simulink model "RoboticsCoursework2"  (R2018b)
settings: Solver=ode4  StartTime=0.0  StopTime=5.0  FixedStep=0.005  RelTol=1e-3
undefined symbols (not defined in the file or in its folder): p560
libraries: roblocks x4
settings Model: Creator=57035  LastModifiedBy=57035

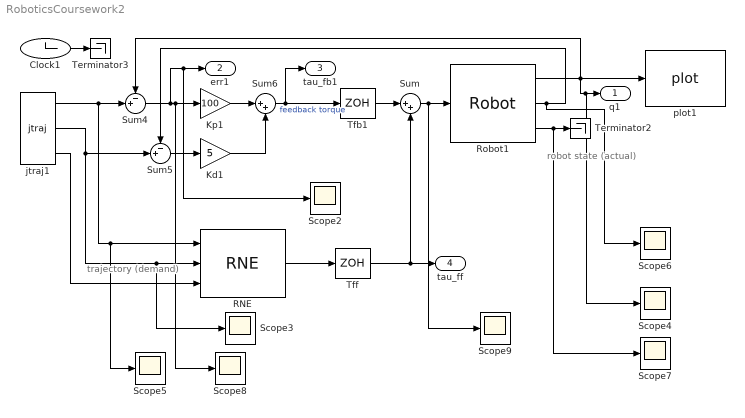
== system RoboticsCoursework2 ==
  note: trajectory
      | (demand)
  note: robot state
      | (actual)
  Clock1 : Clock
  Kd1 : Gain  Gain=5  SaturateOnIntegerOverflow=on  OutDataTypeStr=Inherit: Same as input  ParamDataTypeStr=Inherit: Same as input
  Kp1 : Gain  Gain=100  SaturateOnIntegerOverflow=on  OutDataTypeStr=Inherit: Same as input  ParamDataTypeStr=Inherit: Same as input
  RNE : roblocks/Dynamics/RNE  robot=p560.nofriction()  grav=[0 0 9.81]
  Robot1 : roblocks/Dynamics/Robot  robot=p560  q0=[3.2311 1.9518 0.0224 0 1.1674 -1.4813]
  Scope{2..9} (8 alike) : Scope
  Sum : Sum  Inputs=|++
  Sum4 : Sum  Inputs=-+|  SaturateOnIntegerOverflow=on  InputSameDT=on  OutDataTypeStr=Inherit: Same as first input
  Sum5 : Sum  Inputs=-+|  SaturateOnIntegerOverflow=on  InputSameDT=on  OutDataTypeStr=Inherit: Same as first input
  Sum6 : Sum  Inputs=|++  SaturateOnIntegerOverflow=on  InputSameDT=on  OutDataTypeStr=Inherit: Same as first input
  Terminator2 : Terminator
  Terminator3 : Terminator
  Tfb1 : ZeroOrderHold  SampleTime=0.05
  Tff : ZeroOrderHold  SampleTime=0.05
  jtraj1 : roblocks/Trajectory/jtraj  q0=[3.2311 1.9518 0.0224 0 1.1674 -1.4813]  qf=[3.5865 2.8632 -1.2022 1.6137 1.1278 -1.6707]  tmax=5  ts=0.05
  plot1 : roblocks/Robot Graphics/plot  robot=p560  fps=25  holdplot=on
  q1 : Outport
  err1 : Outport  Port=2
  tau_fb1 : Outport  Port=3
  tau_ff : Outport  Port=4
  wires:
  jtraj1/1 -> Sum4/2, RNE/1, Scope5/1
  Sum6/1 -> Tfb1/1, tau_fb1/1  "feedback torque"
  Kd1/1 -> Sum6/2
  jtraj1/2 -> Sum5/2, Scope3/1, RNE/2
  Sum4/1 -> Scope8/1, Kp1/1, Scope2/1, err1/1
  Kp1/1 -> Sum6/1
  Robot1/3 -> Scope7/1, Terminator2/1
  Robot1/2 -> Scope6/1, Sum5/1
  Sum5/1 -> Kd1/1
  Robot1/1 -> Scope4/1, q1/1, plot1/1, Sum4/1
  Clock1/1 -> Terminator3/1
  RNE/1 -> Tff/1
  jtraj1/3 -> RNE/3
  Tfb1/1 -> Sum/1
  Sum/1 -> Robot1/1, Scope9/1
  Tff/1 -> tau_ff/1, Sum/2
